simulink model "tiltrotor_indi"  (R2024a)
settings: Solver=ode4  StartTime=0.0  StopTime=12  FixedStep=0.0025  RelTol=1e-3
InitFcn:
  | p = tiltrotor_params(); x0_tilt = zeros(19,1); x0_tilt(3) = -50; x0_tilt(7:10) = quat_from_euler(0,0,0); x0_tilt(14:19) = hover_trim(p);
settings Model: Creator=umran  LastModifiedBy=umran

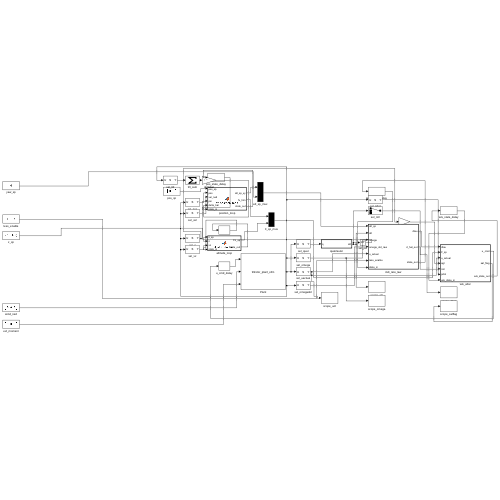
[thumbnail: Simulink's stored preview of the top-level diagram]
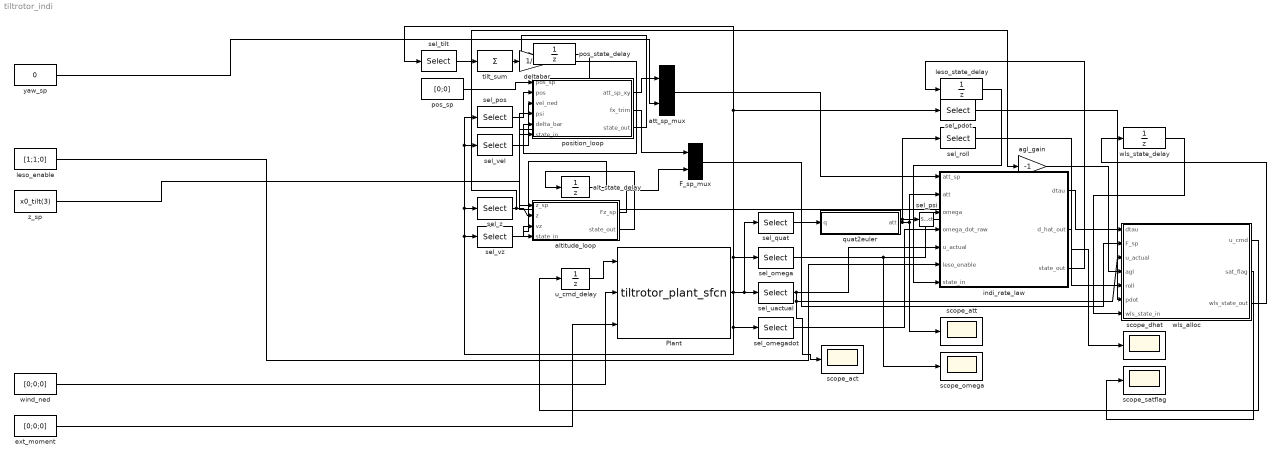
== system tiltrotor_indi ==
  F_sp_mux : Mux  Inputs=2
  Plant : M-S-Function  FunctionName=tiltrotor_plant_sfcn  Parameters=p, x0_tilt
  agl_gain : Gain  Gain=-1
  alt_state_delay : UnitDelay  SampleTime=-1  HasFrameUpgradeWarning=on
  altitude_loop : MATLAB Function  TreatAsAtomicUnit=on
  att_sp_mux : Mux  Inputs=2
  deltabar : Gain  Gain=1/3
  ext_moment : Constant  Value=[0;0;0]
  indi_rate_law : MATLAB Function  TreatAsAtomicUnit=on
  leso_enable : Constant  Value=[1;1;0]
  leso_state_delay : UnitDelay  InitialCondition=zeros(13,1)  SampleTime=-1  HasFrameUpgradeWarning=on
  pos_sp : Constant  Value=[0;0]
  pos_state_delay : UnitDelay  InitialCondition=zeros(2,1)  SampleTime=-1  HasFrameUpgradeWarning=on
  position_loop : MATLAB Function  TreatAsAtomicUnit=on
  quat2euler : MATLAB Function  TreatAsAtomicUnit=on
  scope_act : Scope
  scope_att : Scope
  scope_dhat : Scope
  scope_omega : Scope
  scope_satflag : Scope
  sel_omega : Selector  InputPortWidth=38  IndexOptions=Index vector (dialog)  Indices=11:13  OutputSizes=1
  sel_omegadot : Selector  InputPortWidth=38  IndexOptions=Index vector (dialog)  Indices=30:32  OutputSizes=1
  sel_pdot : Selector  InputPortWidth=38  IndexOptions=Index vector (dialog)  Indices=30  OutputSizes=1
  sel_pos : Selector  InputPortWidth=38  IndexOptions=Index vector (dialog)  Indices=1:2  OutputSizes=1
  sel_psi : Selector  InputPortWidth=3  IndexOptions=Index vector (dialog)  Indices=3  OutputSizes=1
  sel_quat : Selector  InputPortWidth=38  IndexOptions=Index vector (dialog)  Indices=7:10  OutputSizes=1
  sel_roll : Selector  InputPortWidth=3  IndexOptions=Index vector (dialog)  Indices=1  OutputSizes=1
  sel_tilt : Selector  InputPortWidth=38  IndexOptions=Index vector (dialog)  Indices=17:19  OutputSizes=1
  sel_uactual : Selector  InputPortWidth=38  IndexOptions=Index vector (dialog)  Indices=14:19  OutputSizes=1
  sel_vel : Selector  InputPortWidth=38  IndexOptions=Index vector (dialog)  Indices=20:21  OutputSizes=1
  sel_vz : Selector  InputPortWidth=38  IndexOptions=Index vector (dialog)  Indices=22  OutputSizes=1
  sel_z : Selector  InputPortWidth=38  IndexOptions=Index vector (dialog)  Indices=3  OutputSizes=1
  tilt_sum : Sum  Inputs=+
  u_cmd_delay : UnitDelay  InitialCondition=x0_tilt(14:19)  SampleTime=-1  HasFrameUpgradeWarning=on
  wind_ned : Constant  Value=[0;0;0]
  wls_alloc : MATLAB Function  TreatAsAtomicUnit=on
  wls_state_delay : UnitDelay  InitialCondition=zeros(5,1)  SampleTime=-1  HasFrameUpgradeWarning=on
  yaw_sp : Constant  Value=0
  z_sp : Constant  Value=x0_tilt(3)
  wires:
  Plant/1 -> sel_pdot/1, sel_tilt/1, sel_omega/1, sel_vel/1, sel_pos/1, sel_z/1, sel_vz/1, sel_omegadot/1, sel_quat/1, sel_uactual/1
  sel_quat/1 -> quat2euler/1(q)
  att_sp_mux/1 -> indi_rate_law/1(att_sp)
  quat2euler/1(att) -> indi_rate_law/2(att), scope_att/1, sel_psi/1, sel_roll/1
  sel_omega/1 -> indi_rate_law/3(omega), scope_omega/1
  sel_omegadot/1 -> indi_rate_law/4(omega_dot_raw)
  sel_uactual/1 -> wls_alloc/3(u_actual), scope_act/1, indi_rate_law/5(u_actual)
  leso_enable/1 -> indi_rate_law/6(leso_enable)
  leso_state_delay/1 -> indi_rate_law/7(state_in)
  indi_rate_law/3(state_out) -> leso_state_delay/1
  z_sp/1 -> altitude_loop/1(z_sp)
  sel_z/1 -> altitude_loop/2(z), agl_gain/1
  sel_vz/1 -> altitude_loop/3(vz)
  alt_state_delay/1 -> altitude_loop/4(state_in)
  altitude_loop/2(state_out) -> alt_state_delay/1
  position_loop/2(fx_trim) -> F_sp_mux/1
  pos_sp/1 -> position_loop/1(pos_sp)
  sel_pos/1 -> position_loop/2(pos)
  sel_vel/1 -> position_loop/3(vel_ned)
  sel_psi/1 -> position_loop/4(psi)
  sel_tilt/1 -> tilt_sum/1
  tilt_sum/1 -> deltabar/1
  deltabar/1 -> position_loop/5(delta_bar)
  pos_state_delay/1 -> position_loop/6(state_in)
  position_loop/3(state_out) -> pos_state_delay/1
  position_loop/1(att_sp_xy) -> att_sp_mux/1
  yaw_sp/1 -> att_sp_mux/2
  altitude_loop/1(Fz_sp) -> F_sp_mux/2
  indi_rate_law/1(dtau) -> wls_alloc/1(dtau)
  F_sp_mux/1 -> wls_alloc/2(F_sp)
  agl_gain/1 -> wls_alloc/4(agl)
  sel_roll/1 -> wls_alloc/5(roll)
  sel_pdot/1 -> wls_alloc/6(pdot)
  wls_state_delay/1 -> wls_alloc/7(wls_state_in)
  wls_alloc/3(wls_state_out) -> wls_state_delay/1
  wls_alloc/1(u_cmd) -> u_cmd_delay/1
  u_cmd_delay/1 -> Plant/1
  wind_ned/1 -> Plant/2
  ext_moment/1 -> Plant/3
  indi_rate_law/2(d_hat_out) -> scope_dhat/1
  wls_alloc/2(sat_flag) -> scope_satflag/1

== matlab function tiltrotor_indi/indi_rate_law ==
  data: att_sp input; dtau output; att input; omega input; omega_dot_raw input; u_actual input; leso_enable input; state_in input; d_hat_out output; state_out output
function [dtau, d_hat_out, state_out] = sf_indi_rate_law(att_sp, att, omega, omega_dot_raw, u_actual, leso_enable, state_in)
%SF_INDI_RATE_LAW  MATLAB Function blok icerigi: disaridaki attitude P +
%icerideki INDI rate kanunu + LESO bozucu telafisi + basit gain-scheduling.
%#codegen
%
% SAF fonksiyon (persistent YOK) — durum disaridan state_in(13x1) olarak
% girer, state_out(13x1) olarak cikar ve Simulink diyagraminda bir Unit
% Delay ile kendine geri baglanir (bkz. tiltrotor_indi_build.m). Bu, MATLAB
% Function bloklarinin "persistent + surekli ornekleme zamani" kisitini
% (bkz. dosya notu asagida) tamamen ortadan kaldirir.
%
% state_in/out duzeni (13x1): [z1(3); z2(3); prev_u_leso(3); leso_accum(1); omega_dot_filt(3)]
%
% Sabitler tiltrotor_params.m / gain_schedule.m / indi_attitude_controller.m
% ile AYNI degerlerdir (derleme-zamaninda gomulu).

z1            = state_in(1:3);
z2            = state_in(4:6);
prev_u_leso   = state_in(7:9);
leso_accum    = state_in(10);
omega_dot_filt= state_in(11:13);

Ts_ctrl = 0.0025;   % s, 400 Hz — tiltrotor_params.m: p.Ts_ctrl
Ts_leso = 0.005;    % s, 200 Hz — tiltrotor_params.m: p.Ts_leso
I_diag  = [0.2; 0.25; 0.25];

%% --- "Sensor" tarafi: raw turev + tek kutuplu filtre (alpha=0.3) ---
omega_dot_filt = omega_dot_filt + 0.3*(omega_dot_raw - omega_dot_filt);

%% --- Gain-scheduling (ortalama tilt acisina gore, smoothstep) ---
delta_bar = mean(u_actual(4:6));
s = max(0, min(1, delta_bar/(pi/2)));
w = 3*s^2 - 2*s^3;

Kp_att_hover  = [3.0; 3.0; 1.5];
Kp_att_cruise = [2.0; 2.0; 1.0];
Kp_att = Kp_att_hover + (Kp_att_cruise - Kp_att_hover)*w;

Kp_rate_hover  = [4.0; 4.0; 2.0];
Kp_rate_cruise = [3.0; 3.0; 1.5];
Kp_rate = Kp_rate_hover + (Kp_rate_cruise - Kp_rate_hover)*w;

%% --- Disaridaki attitude P dongusu ---
e_att = att_sp - att;
e_att(3) = atan2(sin(e_att(3)), cos(e_att(3)));   % yaw hata sarmalama
% Eksen bazli rate setpoint doygunu (2026-07-27, Adim 13; eskiden skaler 3.0).
% Simulink codegen-safe rewrite oldugu icin p.* yerine literal tutulur --
% tiltrotor_params.m'deki p.ctrl.rate_sp_limit ile AYNI kalmali.
rate_sp_limit = [3.0; 3.0; 0.5];
omega_sp = max(min(Kp_att.*e_att, rate_sp_limit), -rate_sp_limit);

%% --- Ic INDI rate dongusu: istenen acisal ivme ---
e_omega = omega_sp - omega;
omega_dot_des = Kp_rate .* e_omega;

%% --- LESO guncelleme (decimasyonlu, sadece etkin eksenler) ---
d_hat = z2;
leso_accum = leso_accum + Ts_ctrl;
if leso_accum >= Ts_leso - 1e-12
    wo = 15;                 % rad/s, gozlemci bant genisligi
    beta1 = 2*wo;
    beta2 = wo^2;
    for ax = 1:3
        if leso_enable(ax) > 0.5
            e = omega(ax) - z1(ax);
            z1(ax) = z1(ax) + Ts_leso*(z2(ax) + prev_u_leso(ax) + beta1*e);
            z2(ax) = z2(ax) + Ts_leso*(beta2*e);
        end
    end
    d_hat = z2;
    leso_accum = leso_accum - Ts_leso;
end

d_hat_active = d_hat .* leso_enable;
omega_dot_des_adj = omega_dot_des - d_hat_active;

% ESO'nun "girisi": bozucu-telafili (GERCEKTEN uygulanmasi istenen) ivme —
% telafi ONCESI deger kullanilirsa ESO kendi telafisini gormemis gibi
% davranir ve z2 sinirsizca surukler.
prev_u_leso = omega_dot_des_adj;

%% --- INDI artimli kontrol kanunu ---
domega_dot = omega_dot_des_adj - omega_dot_filt;
dtau = I_diag .* domega_dot;

d_hat_out = d_hat;
state_out = [z1; z2; prev_u_leso; leso_accum; omega_dot_filt];

end

== matlab function tiltrotor_indi/quat2euler ==
  data: q input; att output
function att = sf_quat_to_euler(q)
%SF_QUAT_TO_EULER  MATLAB Function blok icerigi: kuaterniyon -> ZYX Euler.
%#codegen
q0=q(1); q1=q(2); q2=q(3); q3=q(4);
phi   = atan2(2*(q0*q1+q2*q3), 1-2*(q1^2+q2^2));
theta = asin(max(-1,min(1, 2*(q0*q2-q3*q1))));
psi   = atan2(2*(q0*q3+q1*q2), 1-2*(q2^2+q3^2));
att = [phi;theta;psi];
end

== matlab function tiltrotor_indi/wls_alloc ==
  data: dtau input; u_cmd output; F_sp input; u_actual input; agl input; roll input; pdot input; wls_state_in input; sat_flag output; wls_state_out output
function [u_cmd, sat_flag, wls_state_out] = sf_wls_alloc(dtau, F_sp, u_actual, ...
                                                         agl, roll, pdot, wls_state_in)
%SF_WLS_ALLOC  MATLAB Function blok icerigi: anlik etkinlik Jacobian'i +
%agirlikli en kucuk kareler (WLS) kontrol tahsisi, kutu-kisitli, + INIS UCLUSU.
%#codegen
%
% effectiveness_matrix.m ile AYNI geometrik model, wls_allocate.m ile ayni
% amac fonksiyonu — ama MATLAB Function blogu icin `find`/degisken-boyutlu
% dizi kullanmadan, sabit-boyutlu "buyuk-M ceza" yontemiyle yeniden yazildi:
% kutu kisitini ihlal eden bir aktuator, kumeden CIKARILMAK yerine agirligi
% asiri buyutulerek (Wu->1e6) o sinira "yapistirilir" — active-set ile ayni
% sonuca yakinsar, degisken boyut gerektirmez.
%
% Girisler:
%   dtau      (3x1 Nm)  INDI moment artisi
%   F_sp      (2x1 N)   istenen govde-eksen [Fx;Fz]
%   u_actual  (6x1)     [T0;T1;T2;d0;d1;d2] aktuator GERCEK durumu
%   agl       (1x1 m)   YERDEN yukseklik -- ham -z DEGIL, bkz. asagidaki not
%   roll      (1x1 rad) olculen roll acisi (temas dalinin ilk olcutu)
%   pdot      (1x1 rad/s^2) olculen roll acisal ivmesi (ikinci temas olcutu)
%   wls_state_in (5x1)  [temas_bekleme_s; temas_mandali(0/1); prev_du_tilt(3)]
% Ciktilar:
%   u_cmd     (6x1)     yeni aktuator komutu (mutlak, [T;delta])
%   sat_flag  (6x1)     0/1, doyuma ulasan aktuatorler
%   wls_state_out (5x1) guncellenmis durum (Unit Delay ile geri baglanir)
%
% YUZEYLER BILEREK YOK (Adim 125): PX4'un UCAN yapilandirmasinda
% SURF_ENABLE = false, yani yuzeyler WLS tahsisatina HIC girmiyor. Iki deneme
% de SITL'de basarisiz oldu ve kayit olarak duruyor (TiltrotorIndiParams.hpp
% SURF_ENABLE basligi: 1. deneme uc rotoru 45 N'e cakti ve seyir tiltini
% 44 -> 13.3 dereceye dusurdu; 2. deneme araci TERS DONDURDU). MATLAB
% referansinin sanal-esleme yaklasimi (Gv = Gp*Mv) PX4'e hic tasinmadi, yani
% SITL'de hic denenmedi. Bu dosya UCAN yapilandirmayi hedefler.

% NOTE (2026-07-26): a Y sign-flip was tried here to match the SDF's
% "right/left" comments and REVERTED -- it caused a ~100-1000x RMS
% regression in the pure-MATLAB reference test. See tiltrotor_params.m note.
% SYNCED with tiltrotor_params.m p.rotor.pos (wing rotors moved above the
% wing, Z 0.06 -> -0.11, 2026-08-16 friend's fix).
rpos = [0.22   0.22  -0.65;
        0.25  -0.25   0.00;
       -0.11  -0.11  -0.07];
% SIGN FIX (2026-07-27, step 12): was [+0.06,-0.06,+0.06]. The magnitude
% matches the SDF <momentConstant> and the (+,-,+) pattern matches the
% ccw/cw/ccw turningDirections, but the OVERALL sign in FRD was inverted:
% gz applies tau_z(FLU) = -turningDirection*T*km, which is +km*T in FRD,
% while this model's m_i = km_i*T_i*dir_i (dir=(0,0,-1)) gives -km*T.
% See tiltrotor_params.m for the full derivation + SITL confirmation.
km = [-0.06, 0.06, -0.06];

T  = u_actual(1:3);
de = u_actual(4:6);

G   = zeros(5,6);
nu0 = zeros(5,1);
for i = 1:3
    s_i = sin(de(i)); c_i = cos(de(i));
    dir_i  = [s_i; 0; -c_i];
    ddir_i = [c_i; 0;  s_i];
    ri = rpos(:,i);

    f_i = T(i)*dir_i;
    m_i = km(i)*T(i)*dir_i;
    tau_i = cross(ri, f_i) + m_i;

    dtau_dT     = cross(ri, dir_i) + km(i)*dir_i;
    dtau_ddelta = (cross(ri, ddir_i) + km(i)*ddir_i) * T(i);

    nu0(1:3) = nu0(1:3) + tau_i;
    nu0(4) = nu0(4) + f_i(1);
    nu0(5) = nu0(5) + f_i(3);

    G(1:3, i)   = dtau_dT;
    G(1:3, 3+i) = dtau_ddelta;
    G(4, i)   = dir_i(1);
    G(4, 3+i) = T(i)*ddir_i(1);
    G(5, i)   = dir_i(3);
    G(5, 3+i) = T(i)*ddir_i(3);
end

%% --- Gain-scheduled WLS agirliklari ---
delta_bar = mean(de);
s = max(0, min(1, delta_bar/(pi/2)));
w = 3*s^2 - 2*s^3;

% NOT (madde (P), Adim 28): Fx trim BURADA uygulanmaz — position_loop.m'de
% uretilip F_sp(1) ile gelir, cunku bedeli olan kalici +Fx'i ancak yatay
% pozisyon dongusu tasiyabilir. Gerekce: indi_attitude_controller.m ayni yer.
dF = F_sp - nu0(4:5);
nu_des = [dtau; dF];

%% --- INIS UCLUSU, 1/3: TEMASTA MOMENT ARTIMI KESILIR (Adim 119) ---
% indi_attitude_controller.m'deki ayni blogun birebir karsiligi.
% Adim 118 olctu ki tek tek CIKIS kanallarini kirpmak sarmayi tahsisatin
% icinde KOVALIYOR: kanat itki farki sifirlaninca ayni sarma tilt kanalina
% gociyor (T0=T1 tam esitken d0/d1 ~4.6 deg/s rampa, tilt farki 7.6 -> 38.1
% deg, yaw kacti). Kusur cikista degil ARTIMDA: yerde omega_dot ~ 0 kaldigi
% icin dtau hic sonmuyor ve WLS onu hangi aktuator ucuzsa oraya biriktiriyor.
%
% YALNIZCA MOMENT: temasta arac agirlik merkezi etrafinda degil TEMAS NOKTASI
% etrafinda doner, yani etkinlik matrisinin moment satirlari o rejimde
% GECERSIZDIR. Kuvvet satirlari gecerlidir; Fz'yi de kesmek irtifa dongusunun
% yerde itkiyi azaltmasini engellerdi.
%
% Mandal BIR ONCEKI tikten gelir (land_state_in), yani degerlendirme bir tik
% gecikmelidir -- referansta da oyle.
land_dwell   = wls_state_in(1);
land_latch   = wls_state_in(2) > 0.5;
prev_du_tilt = wls_state_in(3:5);
if land_latch
    nu_des(1:3) = 0;
end
% wu_tilt_hover=3.0 (was 8.0): keeps tilt cheaper than the ~3.665 threshold
% where WLS starts preferring thrust drain over tilt for roll correction
% -- see gain_schedule.m for the full derivation. NOTE: SITL validation
% (2026-07-26) showed this alone does not fix the T0/T1 lockup, only
% relocates it -- see sitl/RUNBOOK.md "Aday cozum 2".
wu_tilt = 3.0 + (1.5 - 3.0)*w;

% Fx onceligi (4. satir) dusuk: yaw'i duzelten diferansiyel tilt ayni zamanda
% onemli bir Fx uretir; Fx=0'i roll/pitch mertebesinde agirliklandirmak WLS'i
% "sapmayi durdur" ile "Fx=0" arasinda sonlanmayan bir cekismeye sokuyor ve
% delta1 rate-limit sinirinda +/- salinip attitude asla referansa donmuyor.
% Deneysel olarak Ws_Fx ~0.1 altina inince bu cekisme tamamen kalkiyor (bkz.
% indi_attitude_controller.m ayni notu).
% NOTE (2026-07-26): Ws_yaw=6 was tried and REVERTED -- see sitl/RUNBOOK.md
% "Adim 7". It did not help yaw (nu_des(2) barely moved for ~14s, same as
% Ws_yaw=3) and made things worse elsewhere (Fx demand grew to -28N, roll
% grew larger, T0 still collapsed to 0 by the end).
Ws_v = [200; 200; 3; 0.05; 20];
Wu_v = [1; 1; 1; wu_tilt; wu_tilt; wu_tilt*3];

%% --- Kutu kisitlari (mutlak + hiz limiti) ---
Tmin = 0; Tmax = 45; dmin = 0; dmax = pi/2;
tau_up = 0.0125; tau_down = 0.025;
Ts_ctrl = 0.0025;
% AYRISTIRILDI 3.0 -> 4.8 (2026-07-29, Adim 27). Bu sabit artik fiziksel servo
% limiti (p.tilt.rate_max = 3.0, plant clamp'i) DEGIL, yalnizca WLS tahsisat
% kutusudur (p.tilt.slew_box_rate). Codegen-safe olmasi icin literal tutuluyor —
% tiltrotor_params.m'deki p.tilt.slew_box_rate ile SENKRON KALMALI.
% Deger PX4'un tick-basi kutusuna esitlendi: 3.00*(1/250) = 0.012 rad/tick,
% MATLAB 400 Hz'de 0.012/0.0025 = 4.8 rad/s. Gerekce: tiltrotor_params.m.
slew_box_rate_tilt = 4.8;

abs_lo = [Tmin;Tmin;Tmin;dmin;dmin;dmin] - u_actual;
abs_hi = [Tmax;Tmax;Tmax;dmax;dmax;dmax] - u_actual;
rate_lo = [-Tmax/tau_up*Ts_ctrl*5*ones(3,1);   -slew_box_rate_tilt*Ts_ctrl*ones(3,1)];
rate_hi = [ Tmax/tau_down*Ts_ctrl*5*ones(3,1);   slew_box_rate_tilt*Ts_ctrl*ones(3,1)];
du_min = max(abs_lo, rate_lo);
du_max = min(abs_hi, rate_hi);

%% --- TILTJERK (Adim 95/96b) ---
% Slew KUTUSUNUN kendisini KUCULTMEZ -- o, madde (Q)'nun tahsisat acligini
% yeniden acardi (Adim 23/27'de 1.25 -> 3.00 ile kapatilmisti). Bunun yerine
% BIR TUREV USTUNDE calisir: bu tikin du'sunun BIR ONCEKI tikin du'sundan ne
% kadar uzaklasabilecegini sinirlar, yani hiz kutunun bir ucundan digerine tek
% tikte siciramaz.
%
% NEDEN VAR (Adim 94): motor+rotor kutlesini hizla dondurmenin D'Alembert tepki
% torku (I_tilt = 0.01684 kg*m^2) hicbir modelde yok ama Gazebo'nun tam
% cok-cisim fizigi onu otomatik uretiyor -- olculen buyuklugu aktif momentle
% AYNI mertebede (%115). Kontrolcu bunu gormedigi icin kendi kendini besleyen
% bir pitch salinimi olusuyordu.
%
% DEGER: 0.3 rad/s. MATLAB'in ince taramasi 0.25'i onermisti ama GERCEK SITL
% olcumu 0.30'u her metrikte daha iyi buldu (yaw bandi [-4.61,+5.20] vs
% [-7.45,+6.58]; pitch p2p 12.13 vs 15.76 deg) ve karar OLCUME gore verildi
% (Adim 96b). PX4'te de bu deger kalici varsayilandir
% (MulticopterIndiTiltrotor.cpp: _tilt_jerk_limit_mrs = 0.3).
%
% ⚠ REFERANSTAN AYRISIR, BILEREK: indi_attitude_controller.m'de tilt_jerk_limit
% varsayilani Inf'tir (KAPALI) ve yalnizca run_poshold_climb_jerk_sweep.m onu
% veriyor. Bu dosya UCAN yapilandirmayi hedefler (Adim 125), dolayisiyla PX4'un
% varsayilanini alir. Parite testi referansa ayni degeri GECIRIR.
tilt_jerk_limit = 0.3;                      % rad/s
jerk_max = tilt_jerk_limit * Ts_ctrl;
du_min(4:6) = max(du_min(4:6), prev_du_tilt - jerk_max);
du_max(4:6) = min(du_max(4:6), prev_du_tilt + jerk_max);

du_min = min(du_min, du_max);

%% --- Buyuk-M cezali WLS (sabit boyutlu, degisken indeksleme yok) ---
du_pref = zeros(6,1);
Wu_eff  = Wu_v;
big_M   = 1e6;

du = zeros(6,1);
for it = 1:6
    Hm  = G' * (Ws_v.^2 .* G) + diag(Wu_eff.^2);
    rhs = G' * (Ws_v.^2 .* nu_des) + Wu_eff.^2 .* du_pref;
    du  = Hm \ rhs;

    viol_hi = du > du_max;
    viol_lo = du < du_min;
    if ~any(viol_hi) && ~any(viol_lo)
        break;
    end
    du_pref(viol_hi) = du_max(viol_hi);
    du_pref(viol_lo) = du_min(viol_lo);
    Wu_eff(viol_hi | viol_lo) = big_M;
end
du = max(min(du, du_max), du_min);

u_cmd = u_actual + du;
u_cmd(1:3) = max(min(u_cmd(1:3), Tmax), Tmin);

%% --- INIS UCLUSU, 2/3 ve 3/3: KANAT ITKI FARKI SINIRI + TEMAS MANDALI ---
% (Adim 112 sinir, Adim 117 kapinin AGL'si, Adim 118 ikinci temas olcutu.)
% indi_attitude_controller.m ile ayni sirada, ayni sabitlerle.
%
% SABITLER -- tiltrotor_params.m p.ctrl.* ile SENKRON KALMALI (codegen-safe
% olmasi icin literal):
land_diff_max     = 10.0;          % N,   p.ctrl.land_diff_max
land_diff_alt     = 2.0;           % m,   p.ctrl.land_diff_alt
land_contact_roll = 8.0*pi/180;    % rad, p.ctrl.land_contact_roll
land_contact_diff = 6.0;           % N,   p.ctrl.land_contact_diff
land_contact_acc  = 0.05;          % rad/s^2, p.ctrl.land_contact_acc
land_contact_dwl  = 0.20;          % s,   p.ctrl.land_contact_dwell

% KAPI: `agl` YERDEN yukseklik olmak ZORUNDA. Kestirimcinin yerel orijininden
% yukseklik (-z) DEGILDIR -- 23 SITL kosumunda olculen datum ofseti
% -0.67 .. +1.77 m, yani asagidaki 2.0 m'lik esikle AYNI MERTEBEDE. PX4 portu
% Adim 117'ye kadar tam bu hatayi yapiyordu: arac 0.64 m'de yere degdi, sinyal
% 2.41 m dedi, mekanizma hic armanmadi ve fark 45 N'e (tam olcek) gitti.
% tiltrotor_indi_build.m bu porta kalkis datumuna gore duzeltilmis sinyali
% baglar; HAM -z BAGLANMAMALIDIR.
% NaN/Inf korumasi: gecersiz irtifayla kapiyi acmak mekanizmayi ait olmadigi
% bir rejimde devreye sokar; gecersizse KAPALI kalir (PX4'teki alt_ok ile ayni
% guvenli taraf).
if isfinite(agl) && agl < land_diff_alt
    T_mean = 0.5*(u_cmd(1) + u_cmd(2));
    T_diff = 0.5*(u_cmd(1) - u_cmd(2));
    d_lim  = 0.5*land_diff_max;

    % TEMAS DALI 1 -- roll esigi. Olculen TAKLA olayindan (-19.78 deg) turedi;
    % DUZ inisi yakalamaz (orada roll 0.18-0.54 derecede donuyor).
    if abs(roll) > land_contact_roll
        d_lim = 0.0;
    end
    % TEMAS DALI 2 -- mandal (Adim 118). Duz inisi yakalayan dal budur.
    if land_latch
        d_lim = 0.0;
    end

    T_diff = max(min(T_diff, d_lim), -d_lim);
    u_cmd(1) = T_mean + T_diff;
    u_cmd(2) = T_mean - T_diff;
    % Kutuya geri kirp: ortalama kutu icindeyse toplam da icindedir, ama
    % ortalama raya yakinken fark onu disari itebilir.
    u_cmd(1:2) = max(min(u_cmd(1:2), Tmax), Tmin);

    % MANDAL GUNCELLEMESI: "buyuk diferansiyel KOMUT, ama acisal ivme YOK".
    % Serbest ucusta imkansiz -- 6 N, 0.25 m kolda ~1.5 Nm eder ve govdeyi
    % ivmelendirmek zorundadir; yerde zemin momenti karsilar. 26 tam gorev
    % logunda olculen ayrim: AGL > 2 m'de olcut en fazla 0.01 s kesintisiz
    % surdu, AGL < 1.5 m'de 3.28 s'ye kadar. Bekleme suresi o yanlis-pozitifin
    % 20 kati. Mandal SART: fark sifirlaninca olcut kendi kendini bozar ve
    % mandalsiz mekanizma acilip kapanarak salinir.
    if (abs(u_cmd(1) - u_cmd(2)) > land_contact_diff) && (abs(pdot) < land_contact_acc)
        land_dwell = land_dwell + Ts_ctrl;
    else
        land_dwell = 0;
    end
    if land_dwell >= land_contact_dwl
        land_latch = true;
    end
else
    % Kapi kapali (ucus, veya gecersiz irtifa): mandal ve sayac temizlenir --
    % arac 2 m'nin ustune cikinca ucusa donus otomatiktir.
    land_dwell = 0;
    land_latch = false;
end

wls_state_out = [land_dwell; double(land_latch); du(4:6)];

% AYRISMA KAPANDI (Adim 125). Adim 115'ten Adim 124'e kadar bu dosya yere
% yakin itki farki sinirini ICERMIYORDU ve not buraya yazilmisti. Uc mekanizma
% da (Adim 112 sinir, Adim 117 datuma gore AGL, Adim 118 temas mandali,
% Adim 119 artim kesme) yukariya tasindi.
%
% GERIYE KALAN AYRISMALAR (Adim 123 envanteri, bu dosya icin):
%   - fx_trim (Adim 28): F_sp(1) uzerinden gelir, position_loop gerektirir
%   - tiltjerk (Adim 95/96b, 0.3 rad/s): tilt du'suna jerk limiti
%   - ileri/geri gecis, seyir, sabit kanat (Adim 59-103)
% Guncel envanter icin: run_codegen_parity_check
u_cmd(4:6) = max(min(u_cmd(4:6), dmax), dmin);

sat_flag = double(Wu_eff >= big_M);

end

== matlab function tiltrotor_indi/altitude_loop ==
  data: z_sp input; Fz_sp output; z input; vz input; state_in input; state_out output
function [Fz_sp, state_out] = sf_altitude_loop(z_sp, z, vz, state_in)
%SF_ALTITUDE_LOOP  MATLAB Function blok icerigi: basit irtifa dis dongusu
%(P pozisyon + PI hiz, anti-windup) — altitude_loop.m ile ayni mantik,
%persistent yerine SAF fonksiyon + disaridan Unit Delay durum geri beslemesi
%(bkz. sf_indi_rate_law.m'deki ayni desen).
%#codegen
%
% state_in/out (1x1): integral_vz
%
% NOT: pure-MATLAB run_*.m betiklerinde bu dongu Ts_pos=1/50s'de decimasyonlu
% cagrilir (gercekci coklu-hiz mimarisi icin); burada MATLAB Function blogunun
% ayrik ornekleme-zamani ozelligini programatik ayarlamanin guvenilir bir yolu
% bulunamadigi icin (bkz. proje notlari — sf_indi_rate_law'daki persistent
% sorunuyla ayni kok neden), blok her rate-loop adiminda (Ts_ctrl=400 Hz)
% cagriliyor ve Ts asagida ona gore kucultuldu. Matematiksel olarak esdeger
% (integral, ornekleme hizindan bagimsizdir) — sadece CPU'da (ihmal edilebilir
% olsa da) 8 kat daha sik calisir.

m = 5.0; g = 9.81;         % tiltrotor_params.m: p.m, p.g

vz_max = 2.0;
Kp_z   = 0.6;
Kp_vz  = 4.0;
Ki_vz  = 1.5;
int_max = 3.0;

integral_vz = state_in(1);

err_z  = z_sp - z;
vz_sp  = max(min(Kp_z*err_z, vz_max), -vz_max);
err_vz = vz_sp - vz;

Ts_pos = 0.0025; % s, 400 Hz (bkz. yukaridaki not — Ts_ctrl ile ayni cagri hizi)
integral_vz = max(min(integral_vz + err_vz*Ts_pos, int_max), -int_max);

az_corr = Kp_vz*err_vz + Ki_vz*integral_vz;
Fz_sp = m*(az_corr - g);

state_out = integral_vz;

end

== matlab function tiltrotor_indi/position_loop ==
  data: pos_sp input; att_sp_xy output; pos input; vel_ned input; psi input; delta_bar input; state_in input; fx_trim output; state_out output
function [att_sp_xy, fx_trim, state_out] = sf_position_loop(pos_sp, pos, vel_ned, ...
                                                            psi, delta_bar, state_in)
%SF_POSITION_LOOP  MATLAB Function blok icerigi: yatay pozisyon dis dongusu
%(P konum -> PI hiz -> attitude setpoint) + Fx trim.
%#codegen
%
% position_loop.m'in codegen-guvenli yeniden yazimi (Adim 127). AYNI matematik,
% ayni sabitler -- tek fark struct (`p`) yerine literal sabitler ve `state_in`
% ile disaridan gelen durum (MATLAB Function blogu `persistent` kullanamaz).
%
% Girisler:
%   pos_sp   (2x1 m, NED)    istenen yatay konum
%   pos      (2x1 m, NED)    olculen konum
%   vel_ned  (2x1 m/s, NED)  olculen yatay hiz
%   psi      (1x1 rad)       olculen yaw (NED ivmeyi govde-heading'e dondurmek icin)
%   delta_bar(1x1 rad)       ortalama tilt (fx_trim sonumlemesi icin)
%   state_in (2x1 m/s^2)     hiz PI integrali [int_vx; int_vy]
% Ciktilar:
%   att_sp_xy (2x1 rad)      [phi_sp; theta_sp]
%   fx_trim   (1x1 N)        F_sp(1) olarak tahsisata verilecek trim
%   state_out (2x1)          guncellenmis integral
%
% !! BU DONGU YALNIZCA HOVER ICINDIR (Adim 29'da SITL'de aracin dusmesiyle
% ogrenildi). Asagidaki theta_sp = -atan2(ax_b, g) klasik multikopter
% varsayimidir: "yatay kuvvetin tek yolu itki vektorunu egmektir". BU ARACIN
% KANADI VAR. ~5-6 m/s ustunde kanat baskin olur ve burun yukari komutu bir
% FRENLEME degil ENERJI/TIRMANIS komutuna doner. 14.5 m/s'de devreye
% alindiginda olculen: pitch orneklerin %94'unde doydu, hiz 9.6 m/s'de takildi
% ve arac 35 s boyunca ~1.1 m/s tirmandi (z -9.9 -> -54.0 m).
% Dogrulanmis zarf: DURUSTAN devreye alma, <= 3 m/s. PX4 bunu bir kapiyla
% zorlar (POS_ENGAGE_V_MAX); bu blokta kapi YOKTUR, cunku Simulink modeli
% hover senaryosu kosar. Model bir gecis senaryosuna genisletilirse kapi
% EKLENMELIDIR.

% --- SABITLER: position_loop.m ve TiltrotorIndiParams.hpp ile SENKRON KALMALI ---
v_max     = 3.0;            % m/s
Kp_p      = 0.80;           % 1/s
Kp_v      = 2.00;           % (m/s^2)/(m/s)
Ki_v      = 0.40;           % (m/s^2)/(m/s*s)
int_max   = 2.0;            % m/s^2
a_max     = 3.0;            % m/s^2
tilt_max  = 15.0*pi/180;    % rad, govde egim limiti
Ts_pos    = 1/50;           % s,  p.Ts_pos (irtifa dongusuyle ayni decimasyon)
g         = 9.81;           % m/s^2
FX_TRIM   = 2.9;            % N,  p.ctrl.fx_trim / PX4 FX_TRIM
TILT_MAX  = pi/2;           % rad, p.tilt.max (fx_trim sonumlemesinin olcegi)

int_v = state_in(:);

% --- P: konum hatasi -> hiz setpoint'i (NED) ---
err_p = pos_sp(:) - pos(:);
v_sp  = Kp_p * err_p;
nv    = sqrt(v_sp(1)^2 + v_sp(2)^2);    % norm() yerine acik: codegen-guvenli
if nv > v_max
    v_sp = v_sp * (v_max / nv);         % yonu koru, buyuklugu kirp
end

% --- PI: hiz hatasi -> ivme setpoint'i (NED) ---
err_v = v_sp - vel_ned(:);
int_v = int_v + err_v * Ts_pos;
int_v = max(min(int_v, int_max), -int_max);

a_ned = Kp_v * err_v + Ki_v * int_v;
na    = sqrt(a_ned(1)^2 + a_ned(2)^2);
if na > a_max
    a_ned = a_ned * (a_max / na);
end

% --- NED ivme -> govde-heading cercevesi ---
c = cos(psi); s = sin(psi);
ax_b =  a_ned(1)*c + a_ned(2)*s;
ay_b = -a_ned(1)*s + a_ned(2)*c;

% --- ivme -> attitude setpoint ---
theta_sp = -atan2(ax_b, g);
phi_sp   =  atan2(ay_b, g);

theta_sp = max(min(theta_sp, tilt_max), -tilt_max);
phi_sp   = max(min(phi_sp,   tilt_max), -tilt_max);

att_sp_xy = [phi_sp; theta_sp];

% --- Fx TRIM (madde (P), Adim 28) ---
% NEDEN BURADA, tahsisatta DEGIL: tek yonlu tilt araligi ([0, pi/2]) yuzunden
% hover'da Fx >= 0'dir ve yaw trim'i ~2.9 N kalici ileri kuvvet uretir.
% Tahsisattan Fx = 0 istemek, aracin YAPISAL OLARAK iptal edemeyecegi bir
% kuvveti iptal etmesini istemektir.
% Trim dogrudan tahsisata konulursa NE OLUR, olculdu: hover_gust regresyonunda
% q RMS 0.0004 -> 0.0013 (4.3x) kotulesti, cunku o test pozisyon dongusu
% KULLANMIYOR ve olusan ileri kuvveti tasiyacak hicbir sey yok. Bagimlilik
% bu yuzden YAPIYA gomulu: (P) yalnizca (N) aktifken uygulanir. sf_wls_alloc.m
% bu yuzden fx_trim'i KENDI hesaplamaz -- F_sp(1) ile buradan alir.
%
% Gecis boyunca sondurulur (gain_schedule.m ile ayni smoothstep): cruise'da
% tilt zaten buyuk ve Fx kasitli olarak yuksek, orada trim anlamsiz.
s_sched  = max(0, min(1, delta_bar/TILT_MAX));
w_sched  = 3*s_sched^2 - 2*s_sched^3;
fx_trim  = FX_TRIM * (1 - w_sched);

state_out = int_v;

end
